simulink model "s2dot3_46"  (R2023b)
settings: Solver=VariableStepAuto  StartTime=0.0  StopTime=10.0  RelTol=1e-3
settings Model: Creator=lxj  LastModifiedBy=lxj

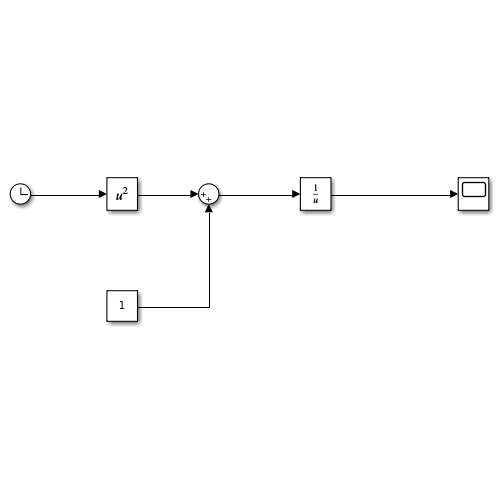
[thumbnail: Simulink's stored preview of the top-level diagram]
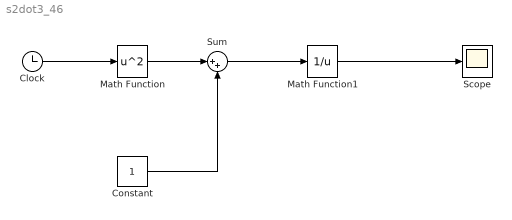
== system s2dot3_46 ==
  Clock : Clock
  Constant : Constant
  Math Function : Math  Operator=square
  Math Function1 : Math  Operator=reciprocal
  Scope : Scope
  Sum : Sum  Inputs=|++
  wires:
  Math Function/1 -> Sum/1
  Sum/1 -> Math Function1/1
  Math Function1/1 -> Scope/1
  Constant/1 -> Sum/2
  Clock/1 -> Math Function/1
